simulink model "coupled_tanks_filtro_wind"  (R2015b)
settings: Solver=ode1  StartTime=0.0  StopTime=100  FixedStep=0.002  RelTol=1e-3
PostLoadFcn:
  | qc_set_target_type(getConfigSet(bdroot, 'QUARC Default Target Configuration'));
undefined symbols (not defined in the file): HIL
libraries: quarc_library x3
settings Model: SimulationMode=external  ExtModeTrigDuration=750000  Creator=MLevis  LastModifiedBy=UFRN
settings SolverCC: PositivePriorityOrder=on
settings DataIOCC: SaveFormat=Array  SignalLoggingSaveFormat=ModelDataLogs
settings OptimizationCC: ExpressionDepthLimit=2147483647  InitFltsAndDblsToZero=on
settings DebuggingCC: SaveWithParameterizedLinksMsg=none  UnderspecifiedInitializationDetection=Classic  MergeDetectMultiDrivingBlocksExec=none  SolverPrmCheckMsg=warning  MultiTaskDSMMsg=warning  MultiTaskCondExecSysMsg=none  FcnCallInpInsideContextMsg=UseLocalSettings  StateNameClashWarn=warning
settings HardwareCC: ProdBitPerPointer=32  ProdLargestAtomicFloat=None  ProdIntDivRoundTo=Undefined  ProdEndianess=Unspecified  ProdWordSize=32  ProdHWDeviceType=32-bit Generic
settings RTWCC: SystemTargetFile=quarc_win64.tlc  TemplateMakefile=quarc_default_tmf  Description=QUARC Win64 Target
settings GRTTargetCC: ParMdlRefBuildCompliant=off  CompOptLevelCompliant=off  GeneratePreprocessorConditionals=Disable all  CombineOutputUpdateFcns=off  MatFileLogging=off  GRTInterface=on  UseToolchainInfoCompliant=off  ExtMode=on  ExtModeMexFile=quarc_comm
settings ConfigComp: CovModelRefEnable=Off

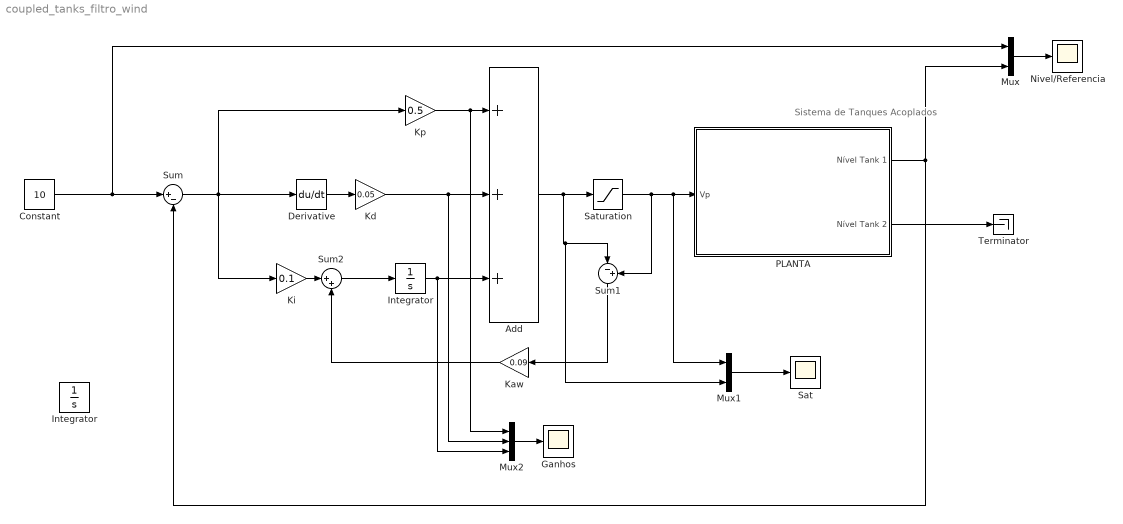
== system coupled_tanks_filtro_wind ==
  note: Sistema de Tanques Acoplados
  Add : Sum  Inputs=+++
  Constant : Constant  Value=10
  Derivative : Derivative
  Ganhos : Scope
  Integrator : Integrator
  "Integrator " : Integrator
  "Kaw " : Gain  Gain=0.09
  "Kd " : Gain  Gain=0.05
  "Ki " : Gain  Gain=0.1
  "Kp " : Gain  Gain=0.5
  Mux : Mux  Inputs=2
  Mux1 : Mux  Inputs=2
  Mux2 : Mux  Inputs=3
  Nivel/Referencia : Scope
  PLANTA : Subsystem
  "Sat " : Scope
  Saturation : Saturate  UpperLimit=4  LowerLimit=-4
  Sum : Sum  Inputs=|+-
  Sum1 : Sum  Inputs=|-+
  Sum2 : Sum  Inputs=|++
  Terminator : Terminator
  wires:
  Sum/1 -> "Ki "/1, Derivative/1, "Kp "/1
  Derivative/1 -> "Kd "/1
  Add/1 -> Mux1/2, Sum1/1, Saturation/1
  Saturation/1 -> Sum1/2, Mux1/1, PLANTA/1(Vp)
  Constant/1 -> Mux/1, Sum/1
  Mux/1 -> Nivel/Referencia/1
  PLANTA/1(Nível Tank 1) -> Mux/2, Sum/2
  Mux1/1 -> "Sat "/1
  Mux2/1 -> Ganhos/1
  "Kp "/1 -> Mux2/1, Add/1
  PLANTA/2(Nível Tank 2) -> Terminator/1
  Sum1/1 -> "Kaw "/1
  "Kd "/1 -> Mux2/2, Add/2
  "Ki "/1 -> Sum2/1
  "Kaw "/1 -> Sum2/2
  Integrator/1 -> Mux2/3, Add/3
  Sum2/1 -> Integrator/1

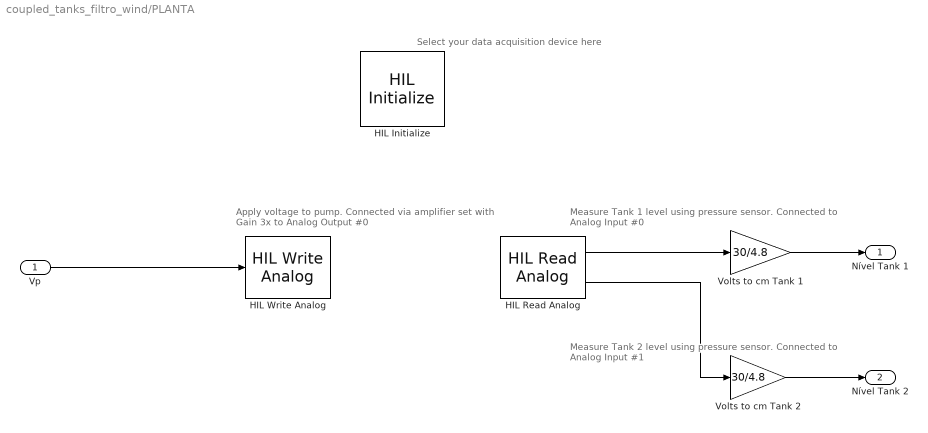
== system coupled_tanks_filtro_wind/PLANTA ==
  note: Select your data acquisition device here
  note: Apply voltage to pump.
      | Connected via amplifier set with Gain 3x
      | to  Analog Output #0
  note: Measure Tank 2 level using pressure sensor.
      | Connected to Analog Input #1
  note: Measure Tank 1 level using pressure sensor.
      | Connected to Analog Input #0
  Vp : Inport
  HIL Initialize : quarc_library/Data Acquisition/Generic/Configuration/HIL Initialize  object_name=HIL-1  board_type=q8_usb  board_number=0  board_options=update_rate=normal;decimation=1  exclusive=off  active=off  hardware_clocks=[0:2]  clock_modes=[]  initial_clock_frequencies=[]  set_clock_params_at_start=off  set_clock_params_at_switch_in=off  set_clock_frequencies_at_start=off  set_clock_frequencies_at_switch_in=off  analog_input_channels=[0:7]  analog_input_maximums=10  analog_input_minimums=-10  set_analog_input_params_at_start=on  set_analog_input_params_at_switch_in=off  analog_output_channels=[0:7]  analog_output_maximums=10  analog_output_minimums=-10  initial_analog_outputs=[0]  final_analog_outputs=[0]  watchdog_analog_outputs=0  set_analog_output_params_at_start=on  set_analog_output_params_at_switch_in=off  set_analog_outputs_at_start=on  set_analog_outputs_at_switch_in=off  set_analog_outputs_at_terminate=on  set_analog_outputs_at_switch_out=off  set_analog_outputs_on_watchdog=off  digital_input_channels=[]  digital_output_channels=[]  digital_output_configuration=[]  initial_digital_outputs=[1]  final_digital_outputs=[1]  watchdog_digital_outputs=[1]  set_digital_output_params_at_start=off  set_digital_output_params_at_switch_in=off  set_digital_outputs_at_start=on  set_digital_outputs_at_switch_in=off  set_digital_outputs_at_terminate=on  set_digital_outputs_at_switch_out=off  set_digital_outputs_on_watchdog=off  encoder_channels=[0:7]  quadrature=[4]  encoder_filter_frequency=[]  initial_encoder_counts=[0]  set_encoder_params_at_start=on  set_encoder_params_at_switch_in=off  set_encoder_counts_at_start=on  set_encoder_counts_at_switch_in=off  pwm_channels=[0:7]  pwm_modes=0  pwm_frequency=99.532799999999995e6/4095  pwm_configuration=[0]  pwm_alignment=[0]  pwm_polarity=[1]  pwm_leading_deadband=[0]  pwm_trailing_deadband=[0]  initial_pwm_outputs=[0]  final_pwm_outputs=[0]  watchdog_pwm_outputs=[0]  set_pwm_params_at_start=on  set_pwm_params_at_switch_in=off  set_pwm_outputs_at_start=on  set_pwm_outputs_at_switch_in=off  set_pwm_outputs_at_terminate=on  set_pwm_outputs_at_switch_out=off  set_pwm_outputs_on_watchdog=off  other_output_channels=[]  initial_other_outputs=[]  final_other_outputs=[]  watchdog_other_outputs=[]  set_other_outputs_at_start=off  set_other_outputs_at_switch_in=off  set_other_outputs_at_terminate=off  set_other_outputs_at_switch_out=off  set_other_outputs_on_watchdog=off
  HIL Read Analog : quarc_library/Data Acquisition/Generic/Immediate I//O/HIL Read Analog  object_name=HIL-1  channels=[0:1]  sample_time=qc_get_step_size  active=on  vector_output=off
  HIL Write Analog : quarc_library/Data Acquisition/Generic/Immediate I//O/HIL Write Analog  object_name=HIL-1  channels=0  sample_time=-1  active=off  vector_input=off
  "Volts to cm Tank 1 " : Gain  Gain=30/4.8
  Volts to cm Tank 2 : Gain  Gain=30/4.8
  Nível Tank 1 : Outport
  Nível Tank 2 : Outport  Port=2
  wires:
  HIL Read Analog/1 -> "Volts to cm Tank 1 "/1
  HIL Read Analog/2 -> Volts to cm Tank 2/1
  Vp/1 -> HIL Write Analog/1
  "Volts to cm Tank 1 "/1 -> Nível Tank 1/1
  Volts to cm Tank 2/1 -> Nível Tank 2/1
